simulink model "RM3"
settings: Solver=ode45  StartTime=0  StopTime=150  FixedStep=0.1  MaxStep=0.1  RelTol=1e-3  EnableMultiTasking=on
undefined symbols (not defined in the file): body, constraint, pto
libraries: WECSim_Lib x5

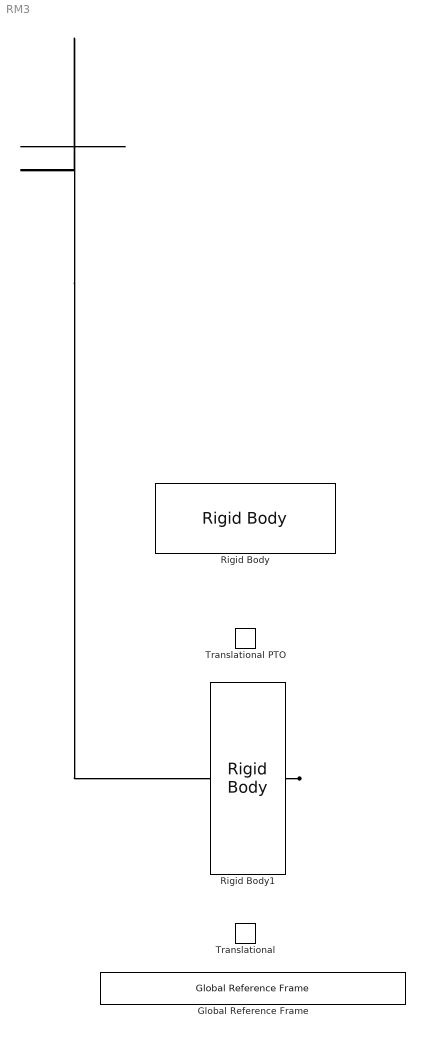
== system RM3 ==
  Global Reference Frame : WECSim_Lib/Frames/Global Reference Frame  waves=waves  simu=simu  waves=waves  simu=simu  waves=waves  simu=simu  waves=waves  simu=simu
  Rigid Body : WECSim_Lib/Body Elements/Rigid Body  body=body(1)  body=body(1)  body=body(1)  body=body(1)
      settings: AttributesFormatString=%<body>
  Rigid Body1 : WECSim_Lib/Body Elements/Rigid Body  body=body(2)  body=body(2)  body=body(2)  body=body(2)
      settings: AttributesFormatString=%<body>
  Translational : WECSim_Lib/Constraints/Translational  constraint=constraint(1)  constraint=constraint(1)  constraint=constraint(1)  constraint=constraint(1)
      settings: AttributesFormatString=%<constraint>
  Translational PTO : WECSim_Lib/PTOs/Translational PTO  pto=pto(1)  pto=pto(1)  pto=pto(1)  pto=pto(1)
      settings: AttributesFormatString=%<pto>
  connections:
  ?
  ?
  ?
